simulink model "MIMO"  (R2019a)
settings: Solver=FixedStepAuto  StartTime=0.0  StopTime=inf  FixedStep=0.00001  RelTol=1e-3
libraries: dsparch4 x10
settings Model: NumberOfSteps=100  Creator=vardhah  LastModifiedBy=vardhah
settings DataIOCC: ReturnWorkspaceOutputs=off
settings DebuggingCC: UnderSpecifiedDimensionMsg=warning  ArithmeticOperatorsInVariantConditions=warning

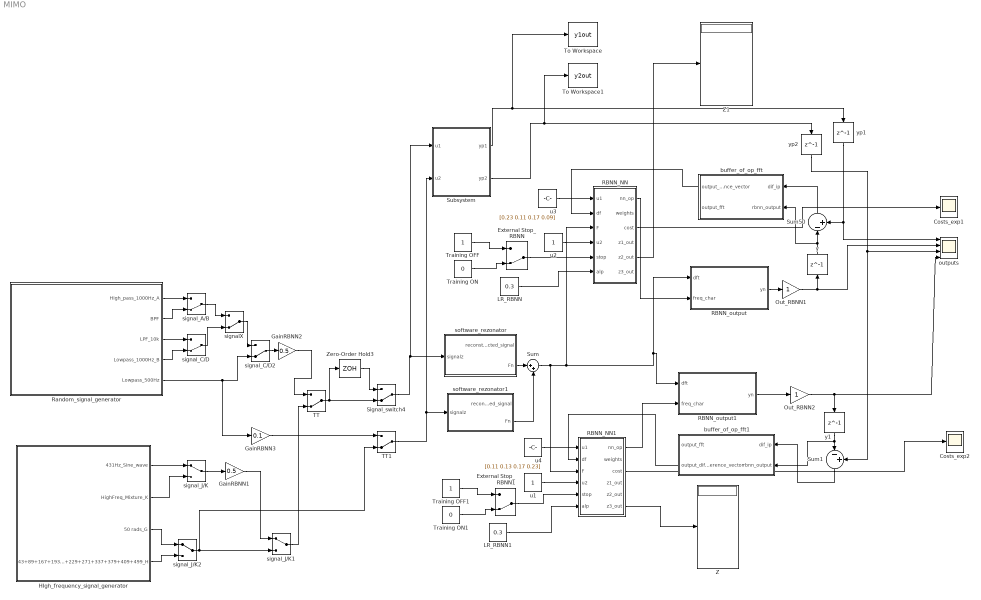
== system MIMO ==
  Costs_exp1 : Scope
  Costs_exp2 : Scope
  External Stop_RBNN : ManualSwitch  CurrentSetting=0
  External Stop_RBNN1 : ManualSwitch  CurrentSetting=0
  GainRBNN1 : Gain  Gain=0.5
  GainRBNN2 : Gain  Gain=0.5
  GainRBNN3 : Gain  Gain=0.1
  HIgh_frequency_signal_generator : Subsystem
  LR_RBNN : Constant  Value=0.3
  LR_RBNN1 : Constant  Value=0.3
  Out_RBNN1 : Gain
  Out_RBNN2 : Gain
  RBNN_NN : MATLAB Function  TreatAsAtomicUnit=on
  RBNN_NN1 : MATLAB Function  TreatAsAtomicUnit=on
  RBNN_output : MATLAB Function  TreatAsAtomicUnit=on
  RBNN_output1 : MATLAB Function  TreatAsAtomicUnit=on
  Random_signal_generator : Subsystem
  Signal_switch4 : ManualSwitch  CurrentSetting=0
  Subsystem : Subsystem
  Sum : Sum  Inputs=|++
  Sum1 : Sum  Inputs=|-+
  Sum50 : Sum  Inputs=|-+
  TT : ManualSwitch  CurrentSetting=0
  TT1 : ManualSwitch  CurrentSetting=0
  To Workspace : ToWorkspace  VariableName=y1out  SampleTime=-1
      settings: Save2DSignal=2-D array (concatenate along first dimension)
  To Workspace1 : ToWorkspace  VariableName=y2out  SampleTime=-1
      settings: Save2DSignal=2-D array (concatenate along first dimension)
  Training OFF : Constant
  Training OFF1 : Constant
  Training ON : Constant  Value=0
  Training ON1 : Constant  Value=0
  Z : Display
  Z1 : Display
  Zero-Order Hold3 : ZeroOrderHold  SampleTime=0.00001
  buffer_of_op_fft : MATLAB Function  TreatAsAtomicUnit=on
  buffer_of_op_fft1 : MATLAB Function  TreatAsAtomicUnit=on
  outputs : Scope  NumInputPorts=4
  signalX : ManualSwitch  CurrentSetting=0
  signal_A/B : ManualSwitch  CurrentSetting=0
  signal_C/D : ManualSwitch  CurrentSetting=0
  signal_C/D2 : ManualSwitch  CurrentSetting=0
  signal_J/K : ManualSwitch
  signal_J/K1 : ManualSwitch
  signal_J/K2 : ManualSwitch
  software_rezonator : MATLAB Function  TreatAsAtomicUnit=on
  software_rezonator1 : MATLAB Function  TreatAsAtomicUnit=on
  u1 : Constant
  u2 : Constant
  u3 : Constant  Value=[0.23 0.11 0.17 0.09]
  u4 : Constant  Value=[0.11 0.13 0.17 0.23]
  y : Delay  DelayLength=1  InitialCondition=0
  y1 : Delay  DelayLength=1  InitialCondition=0
  yp1 : Delay  DelayLength=1  InitialCondition=0
  yp2 : Delay  DelayLength=1  InitialCondition=0
  wires:
  software_rezonator/2(Fn) -> Sum/1
  RBNN_output/1(yn) -> Out_RBNN1/1
  External Stop_RBNN/1 -> RBNN_NN/5(stop)
  Training OFF/1 -> External Stop_RBNN/1
  Training ON/1 -> External Stop_RBNN/2
  Sum50/1 -> buffer_of_op_fft/1(dif_ip)
  TT/1 -> Zero-Order Hold3/1, Signal_switch4/2
  LR_RBNN/1 -> RBNN_NN/6(alp)
  Random_signal_generator/1(High_pass_1000Hz_A) -> signal_A/B/1
  signal_A/B/1 -> signalX/1
  signal_C/D/1 -> signalX/2
  signal_J/K1/1 -> TT/2
  Out_RBNN1/1 -> y/1, outputs/2
  HIgh_frequency_signal_generator/1(431Hz_Sine_wave) -> signal_J/K/1
  HIgh_frequency_signal_generator/2(HighFreq_Mixture_K) -> signal_J/K/2
  signal_J/K/1 -> GainRBNN1/1
  Signal_switch4/1 -> Subsystem/1(u1), software_rezonator/1(signalz)
  Random_signal_generator/3(LPF_10k) -> signal_C/D/1
  Random_signal_generator/2("BPF ") -> signal_A/B/2
  signalX/1 -> signal_C/D2/1
  Random_signal_generator/5(Lowpass_500Hz) -> GainRBNN3/1, signal_C/D2/2
  HIgh_frequency_signal_generator/3(50 rads_G) -> signal_J/K2/1
  HIgh_frequency_signal_generator/4(43+89+167+193+229+271+337+379+409+499_H) -> signal_J/K2/2
  GainRBNN1/1 -> signal_J/K1/1
  signal_C/D2/1 -> GainRBNN2/1
  GainRBNN2/1 -> TT/1
  Zero-Order Hold3/1 -> Signal_switch4/1
  u2/1 -> RBNN_NN/4(u2)
  LR_RBNN1/1 -> RBNN_NN1/6(alp)
  Training ON1/1 -> External Stop_RBNN1/2
  External Stop_RBNN1/1 -> RBNN_NN1/5(stop)
  Training OFF1/1 -> External Stop_RBNN1/1
  u1/1 -> RBNN_NN1/4(u2)
  software_rezonator1/2(Fn) -> Sum/2
  Random_signal_generator/4(Lowpass_1000Hz_B) -> signal_C/D/2
  TT1/1 -> Subsystem/2(u2), software_rezonator1/1(signalz)
  RBNN_NN/1(nn_op) -> RBNN_output/2(freq_char)
  Subsystem/1(yp1) -> To Workspace/1, yp1/1
  buffer_of_op_fft/1(output_difference_vector) -> RBNN_NN/2(df)
  RBNN_NN1/1(nn_op) -> RBNN_output1/2(freq_char)
  buffer_of_op_fft1/2(output_difference_vector) -> RBNN_NN1/2(df)
  y/1 -> buffer_of_op_fft/2(rbnn_output), Sum50/1
  yp1/1 -> outputs/1, Sum50/2
  RBNN_output1/1(yn) -> Out_RBNN2/1
  Out_RBNN2/1 -> y1/1, outputs/4
  Subsystem/2(yp2) -> To Workspace1/1, yp2/1
  yp2/1 -> outputs/3, Sum1/2
  RBNN_NN/3(cost) -> Costs_exp1/1
  Sum1/1 -> buffer_of_op_fft1/1(dif_ip)
  y1/1 -> buffer_of_op_fft1/2(rbnn_output), Sum1/1
  RBNN_NN1/3(cost) -> Costs_exp2/1
  signal_J/K2/1 -> TT1/2, signal_J/K1/2
  RBNN_NN/5(z2_out) -> Z1/1
  Sum/1 -> RBNN_NN1/3(F), RBNN_NN/3(F), RBNN_output/1(dft), RBNN_output1/1(dft)
  GainRBNN3/1 -> TT1/1
  RBNN_NN1/6(z3_out) -> Z/1
  u3/1 -> RBNN_NN/1(u1)
  u4/1 -> RBNN_NN1/1(u1)

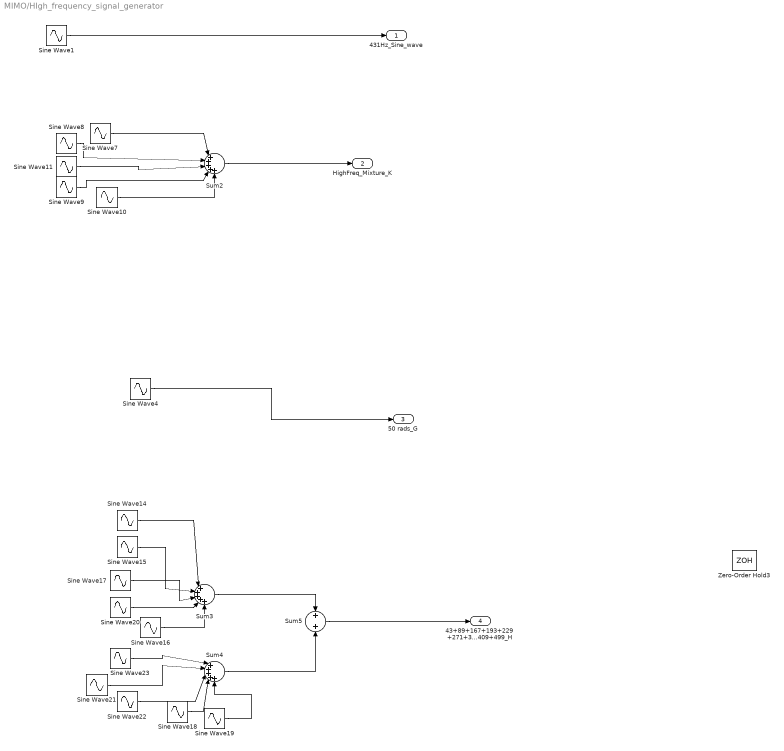
== system MIMO/HIgh_frequency_signal_generator ==
  Sine Wave1 : Sin  Amplitude=0.5  Frequency=431  SampleTime=0
  Sine Wave10 : Sin  Amplitude=2  Frequency=47000  SampleTime=0
  Sine Wave11 : Sin  Amplitude=2  Frequency=30637  SampleTime=0
  Sine Wave14 : Sin  Amplitude=0.1  Frequency=43  SampleTime=0
  Sine Wave15 : Sin  Amplitude=0.1  Frequency=89  SampleTime=0
  Sine Wave16 : Sin  Amplitude=0.1  Frequency=229  SampleTime=0
  Sine Wave17 : Sin  Amplitude=0.1  Frequency=167  SampleTime=0
  Sine Wave18 : Sin  Amplitude=0.1  Frequency=409  SampleTime=0
  Sine Wave19 : Sin  Amplitude=0.1  Frequency=499  SampleTime=0
  Sine Wave20 : Sin  Amplitude=0.1  Frequency=193  SampleTime=0
  Sine Wave21 : Sin  Amplitude=0.1  Frequency=337  SampleTime=0
  Sine Wave22 : Sin  Amplitude=0.1  Frequency=379  SampleTime=0
  Sine Wave23 : Sin  Amplitude=0.1  Frequency=271  SampleTime=0
  Sine Wave4 : Sin  Amplitude=0.5  Frequency=50  SampleTime=0
  Sine Wave7 : Sin  Amplitude=2  Frequency=28230  SampleTime=0
  Sine Wave8 : Sin  Amplitude=2  Frequency=33927  SampleTime=0
  Sine Wave9 : Sin  Amplitude=0  Frequency=53787  SampleTime=0
  Sum2 : Sum  Inputs=|+++++
  Sum3 : Sum  Inputs=|+++++
  Sum4 : Sum  Inputs=|+++++
  Sum5 : Sum
  Zero-Order Hold3 : ZeroOrderHold  SampleTime=0.00001
  431Hz_Sine_wave : Outport
  HighFreq_Mixture_K : Outport  Port=2
  50 rads_G : Outport  Port=3
  43+89+167+193+229+271+337+379+409+499_H : Outport  Port=4
  wires:
  Sine Wave9/1 -> Sum2/4
  Sine Wave7/1 -> Sum2/1
  Sine Wave10/1 -> Sum2/5
  Sine Wave8/1 -> Sum2/2
  Sine Wave11/1 -> Sum2/3
  Sine Wave1/1 -> 431Hz_Sine_wave/1
  Sum2/1 -> HighFreq_Mixture_K/1
  Sine Wave23/1 -> Sum4/1
  Sine Wave17/1 -> Sum3/3
  Sine Wave22/1 -> Sum4/3
  Sine Wave18/1 -> Sum4/4
  Sine Wave19/1 -> Sum4/5
  Sine Wave20/1 -> Sum3/4
  Sine Wave14/1 -> Sum3/1
  Sine Wave15/1 -> Sum3/2
  Sine Wave21/1 -> Sum4/2
  Sine Wave16/1 -> Sum3/5
  Sum4/1 -> Sum5/2
  Sum3/1 -> Sum5/1
  Sine Wave4/1 -> 50 rads_G/1
  Sum5/1 -> 43+89+167+193+229+271+337+379+409+499_H/1

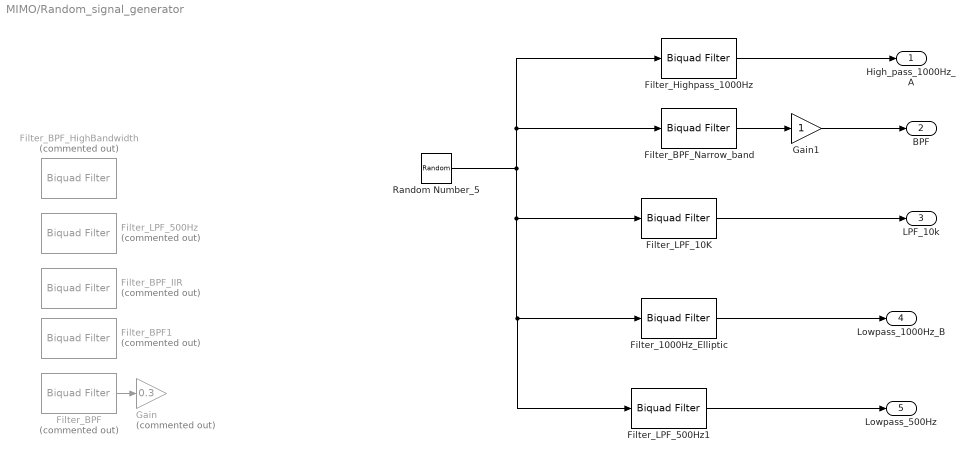
== system MIMO/Random_signal_generator ==
  Filter_1000Hz_Elliptic : dsparch4/Biquad Filter  Tag=BlockMethodSubSystem  FilterSource=Dialog parameters  CoeffSource=Specify via dialog  FilterObject=BQF  IIRFiltStruct=Direct form II  BiQuadCoeffs=[1 -1.97632274641133088 1 1 -1.97939835930391728 0.996447647782941925;1 -1.97278944538463175 1 1 -1.97237302925889701 0.987301248342435933;1 -1.95955871016892758 1 1 -1.96235771308246942 0.972660421241710926;1 -1.88453112329299022 1 1 -1.95007892273323602 0.954154972801176005;1 1 0 1 -0.971866907997287366 0]  ScaleValues=[0.156742012624585314;0.548618699418480849;0.254757160374388947;0.035299988916345823;0.064621492680459483;1]  IC=0  ICnum=0  ICden=0  a0Flag=Warning  optimizeScaleValues=on  ScaleValueMode=Specify via input port (g)  InputProcessing=Columns as channels (frame based)  roundingMode=Floor  overflowMode=off  scaleValueFracLength=14  denProdOutputFracLength=30  denAccumFracLength=30  secondMemoryFracLength=15
      settings: SourceProductName=DSP System Toolbox
  Filter_BPF : dsparch4/Biquad Filter  Tag=BlockMethodSubSystem  Commented=on  FilterSource=Dialog parameters  CoeffSource=Specify via dialog  FilterObject=BQF  IIRFiltStruct=Direct form II  BiQuadCoeffs=[1 -1.97761973100167809 1 1 1.57870632394964705 0.920020418344257962;1 1.77936221516677162 1 1 -1.93552590907125399 0.972267372386662942;1 -1.98005309158266063 1 1 1.47905907116838886 0.778576723939160997;1 1.80228019362095471 1 1 -1.8859717379982055 0.919695136491283316;1 -1.98441806776151775 1 1 -1.84268162877499142 0.871961176321420783;1 1.84402260102226045 1 1 1.40847943705151635 0.659380286133449012;1 -1.98978059787965811 1 1 -1.8064582693224005 0.83068683784082864;1 1.89644656024463654 1 1 1.35993304577530516 0.561880786756156714;1 -1.99493211957147487 1 1 -1.77859151837716212 0.798148234549097224;1 1.94803425022672294 1 1 1.32826652221219343 0.488041230314220198;1 -1.99864670422051782 1 1 -1.76078971043777521 0.777037775895594751;1 1.98600294595924809 1 1 1.31027557706720854 0.441399359096070587;1 0 -1 1 -0.225108906907530854 -0.5721944072401276]  ScaleValues=[0.94218659324992049;0.94218659324992049;0.896412139345828973;0.896412139345828973;0.858240609492223139;0.858240609492223139;0.827592837896180988;0.827592837896180988;0.804900029269587591;0.804900029269587591;0.790860073802791552;0.790860073802791552;0.786097203620063856;1]  IC=0  ICnum=0  ICden=0  a0Flag=Warning  optimizeScaleValues=on  ScaleValueMode=Specify via input port (g)  InputProcessing=Columns as channels (frame based)  roundingMode=Floor  overflowMode=off  scaleValueFracLength=14  denProdOutputFracLength=30  denAccumFracLength=30  secondMemoryFracLength=15
      settings: SourceProductName=DSP System Toolbox
  Filter_BPF1 : dsparch4/Biquad Filter  Tag=BlockMethodSubSystem  Commented=on  FilterSource=Dialog parameters  CoeffSource=Specify via dialog  FilterObject=BQF  IIRFiltStruct=Direct form II  BiQuadCoeffs=[1 -1.87162275664653865 1 1 0.0151789185122153114 0.97249456913610377;1 0.107053815110264378 1 1 -1.8502247355910888 0.989791248656434752;1 -1.87399697860168635 1 1 0.0292079264951085604 0.918601061350948767;1 0.126268370493222148 1 1 -1.83332118307014369 0.969469007130600025;1 -1.87872867044463465 1 1 0.0569157635014451713 0.864412592104086164;1 0.165552966551231862 1 1 -1.81812689818783735 0.948927647744083225;1 -1.88577621884367863 1 1 -1.8041786729911804 0.927783166166077922;1 0.226641198999771337 1 1 0.097812015244096856 0.808034579697935573;1 -1.89505605753386197 1 1 -1.79101562259146441 0.90569591944563943;1 0.312164718875241609 1 1 0.151460725355784309 0.74780602813150221;1 -1.90641512361342702 1 1 -1.77818269270842544 0.882393193837985756;1 0.425602178644961193 1 1 0.217201621241827264 0.682338033780143238;1 -1.91959159061561468 1 1 -1.76525054298619066 0.857713442273093762;1 0.571003956082658304 1 1 0.293797239380520436 0.610677959292126982;1 -1.93416461417083374 1 1 -1.75186392449751338 0.831683197854011347;1 0.752181231021604835 1 1 0.379002473503964599 0.532637148822792561;1 -1.94949927666361944 1 1 -1.73783535618849294 0.804640333462611768;1 0.970805587395975667 1 1 0.469112491907584639 0.449311075928955861;1 -1.96470348628740155 1 1 -1.72330128044392006 0.777413997776565835;1 1.22267124909860003 1 1 0.558648874108559568 0.363760367241365734;1 -1.97862850586430206 1 1 -1.70893825597331972 0.751545290116931608;1 1.49181652406040532 1 1 0.640463654393117032 0.28166537946727177;1 -1.98995570459027227 1 1 -1.6961607248116688 0.729445514574812215;1 1.74459803428737614 1 1 0.706553803150463011 0.211486877483081787;1 -1.9973994069383596 1 1 -1.68705750203480132 0.71421185466085324;1 1.93071581234363698 1 1 0.749581571245088285 0.163359895205374334;1 0 -1 1 -0.45960409018619558 -0.321805205203900269]  ScaleValues=[0.947999620287395151;0.947999620287395151;0.929748841120282554;0.929748841120282554;0.910904712958650942;0.910904712958650942;0.890940239596866634;0.890940239596866634;0.869397912584866428;0.869397912584866428;0.845915862145971476;0.845915862145971476;0.820293089159258471;0.820293089159258471;0.792605314952226081;0.792605314952226081;0.763377121832675587;0.763377121832675587;0.733791113440760645;0.733791113440760645;0.705857588574427597;0.705857588574427597;0.682382892583755729;0.682382892583755729;0.666528818859254413;0.666528818859254413;0.660902602601950107;1]  IC=0  ICnum=0  ICden=0  a0Flag=Warning  optimizeScaleValues=on  ScaleValueMode=Specify via input port (g)  InputProcessing=Columns as channels (frame based)  roundingMode=Floor  overflowMode=off  scaleValueFracLength=14  denProdOutputFracLength=30  denAccumFracLength=30  secondMemoryFracLength=15
      settings: SourceProductName=DSP System Toolbox
  Filter_BPF_HighBandwidth : dsparch4/Biquad Filter  Tag=BlockMethodSubSystem  Commented=on  FilterSource=Dialog parameters  CoeffSource=Specify via dialog  FilterObject=BQF  IIRFiltStruct=Direct form II  BiQuadCoeffs=[1 1.7667446216002245 1 1 1.58209736682341973 0.930966785022698806;1 -1.34582318986797533 1 1 -0.992426842776809148 0.899039050324202504;1 1.79067372195770425 1 1 -0.914728053198516244 0.716995181890824007;1 -1.40612551986482726 1 1 1.48400011430024925 0.801184577292333389;1 1.83602350074132281 1 1 -0.851515418032590565 0.547239550845750156;1 -1.52433209950181525 1 1 1.39252668353121223 0.674238480546462959;1 1.89581887946284833 1 1 1.29703137445886307 0.544576166858187882;1 -1.6885603993121634 1 1 -0.786012220300839282 0.382455837322811409;1 1.95573661837008239 1 1 1.19088356295662234 0.413755766632151967;1 -1.86350238128714696 1 1 -0.705134792353248718 0.2271878178236309;1 1.99461273858363541 1 1 1.09074964949811615 0.306078291590546059;1 -1.98303965563176376 1 1 -0.619529972182138677 0.110169074458665181]  ScaleValues=[0.832448302986908639;0.832448302986908639;0.765789381177460982;0.765789381177460982;0.705208129127222416;0.705208129127222416;0.651112560595629053;0.651112560595629053;0.608221202899987934;0.608221202899987934;0.583850801160644806;0.583850801160644806;1]  IC=0  ICnum=0  ICden=0  a0Flag=Warning  optimizeScaleValues=on  ScaleValueMode=Specify via input port (g)  InputProcessing=Columns as channels (frame based)  roundingMode=Floor  overflowMode=off  scaleValueFracLength=14  denProdOutputFracLength=30  denAccumFracLength=30  secondMemoryFracLength=15
      settings: SourceProductName=DSP System Toolbox
  Filter_BPF_IIR : dsparch4/Biquad Filter  Tag=BlockMethodSubSystem  Commented=on  FilterSource=Dialog parameters  CoeffSource=Specify via dialog  FilterObject=BQF  IIRFiltStruct=Direct form II  BiQuadCoeffs=[1 -1.149490264419329 1 1 -0.626392877901499556 0.920117434054556482;1 0.646230741294248623 1 1 0.0366640948662285138 0.915703951328018961;1 -1.34532900218332485 1 1 -0.519313485606232472 0.780807553044220226;1 0.918145007146928704 1 1 -0.0338871305922869778 0.772019964264916481;1 -1.83355458637284285 1 1 -0.358020160863192105 0.687764548138794729;1 1.69599580965141206 1 1 -0.17451489355262309 0.683094681391207548]  ScaleValues=[0.380605401112502073;0.380605401112502073;0.290603776410566172;0.290603776410566172;0.185292453644045008;0.185292453644045008;1]  IC=0  ICnum=0  ICden=0  a0Flag=Warning  optimizeScaleValues=on  ScaleValueMode=Specify via input port (g)  InputProcessing=Columns as channels (frame based)  roundingMode=Floor  overflowMode=off  scaleValueFracLength=14  denProdOutputFracLength=30  denAccumFracLength=30  secondMemoryFracLength=15
      settings: SourceProductName=DSP System Toolbox
  Filter_BPF_Narrow_band : dsparch4/Biquad Filter  Tag=BlockMethodSubSystem  FilterSource=Dialog parameters  CoeffSource=Specify via dialog  FilterObject=BQF  IIRFiltStruct=Direct form II  BiQuadCoeffs=[1 0.62090288091487722 1 1 0.531418224661316274 0.980919730652416666;1 0.123603302701670317 1 1 0.212906146103049365 0.980314531399748446;1 0.646038601655443578 1 1 0.517597147874857333 0.941099448368431624;1 0.0957486348882208987 1 1 0.211835114073677666 0.93930845670321006;1 0.711459208664077192 1 1 0.494162772086789159 0.895904757499573212;1 0.0218734686284944163 1 1 0.218844224698679646 0.893061304454884519;1 0.877256774030408248 1 1 0.450892485812207533 0.84715521652707737;1 -0.17476459239363229 1 1 0.245263071402918309 0.844050263048180871;1 1.47045699040561728 1 1 0.381616270905086485 0.810187489215232537;1 -1.01162752930746769 1 1 0.302620729086598206 0.808716245866266337]  ScaleValues=[0.644925573949283848;0.644925573949283848;0.594784290548588279;0.594784290548588279;0.499322257310351236;0.499322257310351236;0.34838267808004042;0.34838267808004042;0.155186261234775053;0.155186261234775053;1]  IC=0  ICnum=0  ICden=0  a0Flag=Warning  optimizeScaleValues=on  ScaleValueMode=Specify via input port (g)  InputProcessing=Columns as channels (frame based)  roundingMode=Floor  overflowMode=off  scaleValueFracLength=14  denProdOutputFracLength=30  denAccumFracLength=30  secondMemoryFracLength=15
      settings: SourceProductName=DSP System Toolbox
  Filter_Highpass_1000Hz : dsparch4/Biquad Filter  Tag=BlockMethodSubSystem  FilterSource=Dialog parameters  CoeffSource=Specify via dialog  FilterObject=BQF  IIRFiltStruct=Direct form II  BiQuadCoeffs=[1 -1.9832348135082305 1 1 -1.92871230100246671 0.962722433368264241;1 -1.98583197848424597 1 1 -1.86448430214602556 0.894880266245439038;1 -1.99020937824944788 1 1 -1.81348943480495617 0.839000119522318677;1 -1.99498360843622446 1 1 -1.77690733715439997 0.797591087467987903;1 -1.99863653257112794 1 1 -1.75501257669195576 0.772196386514157451;1 -1 0 1 -0.873867637211059756 0]  ScaleValues=[0.976953385016072651;0.943181897451958351;0.915362881516173843;0.894746706112661938;0.882102920451765637;0.936933818605529933;1]  IC=0  ICnum=0  ICden=0  a0Flag=Warning  optimizeScaleValues=on  ScaleValueMode=Specify via input port (g)  InputProcessing=Columns as channels (frame based)  roundingMode=Floor  overflowMode=off  scaleValueFracLength=14  denProdOutputFracLength=30  denAccumFracLength=30  secondMemoryFracLength=15
      settings: SourceProductName=DSP System Toolbox
  Filter_LPF_10K : dsparch4/Biquad Filter  Tag=BlockMethodSubSystem  FilterSource=Dialog parameters  CoeffSource=Specify via dialog  FilterObject=BQF  IIRFiltStruct=Direct form II  BiQuadCoeffs=[1 2 1 1 -0.612485417634850315 0.975058739649728001;1 2 1 1 -0.698043577421757266 0.925601996299419083;1 2 1 1 -0.874476472259565263 0.875096533006947785;1 2 1 1 -1.12129625964924906 0.823722261210925066;1 2 1 1 -1.39397155012670271 0.77557292582325299;1 2 1 1 -1.61651585106992179 0.739432707187852145;1 1 0 1 -0.851908249730889411 0]  ScaleValues=[0.340643330503719421;0.306889604719415399;0.250155015186845686;0.175606500390419001;0.0954003439241375567;0.0307292140294825808;0.0740458751345553223;1]  IC=0  ICnum=0  ICden=0  a0Flag=Warning  optimizeScaleValues=on  ScaleValueMode=Specify via input port (g)  InputProcessing=Columns as channels (frame based)  roundingMode=Floor  overflowMode=off  scaleValueFracLength=14  denProdOutputFracLength=30  denAccumFracLength=30  secondMemoryFracLength=15
      settings: SourceProductName=DSP System Toolbox
  Filter_LPF_500Hz : dsparch4/Biquad Filter  Tag=BlockMethodSubSystem  Commented=on  FilterSource=Dialog parameters  CoeffSource=Specify via dialog  FilterObject=BQF  IIRFiltStruct=Direct form II  BiQuadCoeffs=[1 -1.99378181081805117 1 1 -1.98902831364610422 0.9935124525991188;1 -1.99333638931724444 1 1 -1.97523846334044983 0.979918343946878045;1 -1.99230894289473004 1 1 -1.95902587969734232 0.964154555843562355;1 -1.99032724021591334 1 1 -1.93837876272327003 0.944275888371317706;1 -1.98644110500488824 1 1 -1.91073325330636345 0.917824821659265599;1 -1.97784207285711422 1 1 -1.87346681472727061 0.882295849747020466;1 -1.95323474003079056 1 1 -1.82673924270665844 0.837830591019173787;1 -1.8251127117585888 1 1 -1.78083961390105383 0.794192376902756902;1 1 0 1 -0.880096604509032043 0]  ScaleValues=[0.721132603368186742;0.702304025434590584;0.6668363107986508;0.609663196407451258;0.523019638064808889;0.398459430018688054;0.237170675835394501;0.0763506778335484859;0.0599516977454839714;1]  IC=0  ICnum=0  ICden=0  a0Flag=Warning  optimizeScaleValues=on  ScaleValueMode=Specify via input port (g)  InputProcessing=Columns as channels (frame based)  roundingMode=Floor  overflowMode=off  scaleValueFracLength=14  denProdOutputFracLength=30  denAccumFracLength=30  secondMemoryFracLength=15
      settings: SourceProductName=DSP System Toolbox
  Filter_LPF_500Hz1 : dsparch4/Biquad Filter  Tag=BlockMethodSubSystem  FilterSource=Dialog parameters  CoeffSource=Specify via dialog  FilterObject=BQF  IIRFiltStruct=Direct form II  BiQuadCoeffs=[1 -1.99378181081805117 1 1 -1.98902831364610422 0.9935124525991188;1 -1.99333638931724444 1 1 -1.97523846334044983 0.979918343946878045;1 -1.99230894289473004 1 1 -1.95902587969734232 0.964154555843562355;1 -1.99032724021591334 1 1 -1.93837876272327003 0.944275888371317706;1 -1.98644110500488824 1 1 -1.91073325330636345 0.917824821659265599;1 -1.97784207285711422 1 1 -1.87346681472727061 0.882295849747020466;1 -1.95323474003079056 1 1 -1.82673924270665844 0.837830591019173787;1 -1.8251127117585888 1 1 -1.78083961390105383 0.794192376902756902;1 1 0 1 -0.880096604509032043 0]  ScaleValues=[0.721132603368186742;0.702304025434590584;0.6668363107986508;0.609663196407451258;0.523019638064808889;0.398459430018688054;0.237170675835394501;0.0763506778335484859;0.0599516977454839714;1]  IC=0  ICnum=0  ICden=0  a0Flag=Warning  optimizeScaleValues=on  ScaleValueMode=Specify via input port (g)  InputProcessing=Columns as channels (frame based)  roundingMode=Floor  overflowMode=off  scaleValueFracLength=14  denProdOutputFracLength=30  denAccumFracLength=30  secondMemoryFracLength=15
      settings: SourceProductName=DSP System Toolbox
  Gain : Gain  Commented=on  Gain=0.3
  Gain1 : Gain
  Random Number_5 : RandomNumber  Variance=0.5  SampleTime=0.00001
  High_pass_1000Hz_A : Outport
  "BPF " : Outport  Port=2
  LPF_10k : Outport  Port=3
  Lowpass_1000Hz_B : Outport  Port=4
  Lowpass_500Hz : Outport  Port=5
  wires:
  Filter_Highpass_1000Hz/1 -> High_pass_1000Hz_A/1
  Filter_1000Hz_Elliptic/1 -> Lowpass_1000Hz_B/1
  Filter_BPF/1 -> Gain/1
  Gain1/1 -> "BPF "/1
  Filter_LPF_10K/1 -> LPF_10k/1
  Random Number_5/1 -> Filter_LPF_500Hz1/1, Filter_1000Hz_Elliptic/1, Filter_LPF_10K/1, Filter_BPF_Narrow_band/1, Filter_Highpass_1000Hz/1
  Filter_BPF_Narrow_band/1 -> Gain1/1
  Filter_LPF_500Hz1/1 -> Lowpass_500Hz/1

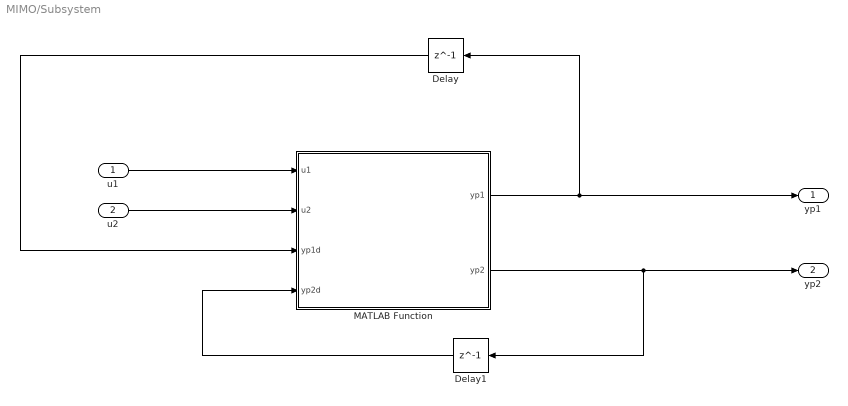
== system MIMO/Subsystem ==
  u1 : Inport
  u2 : Inport  Port=2
  Delay : Delay  DelayLength=1  InitialCondition=0
  Delay1 : Delay  DelayLength=1  InitialCondition=0
  MATLAB Function : MATLAB Function  TreatAsAtomicUnit=on
  yp1 : Outport
  yp2 : Outport  Port=2
  wires:
  u1/1 -> MATLAB Function/1(u1)
  MATLAB Function/2(yp2) -> yp2/1, Delay1/1
  u2/1 -> MATLAB Function/2(u2)
  MATLAB Function/1(yp1) -> Delay/1, yp1/1
  Delay/1 -> MATLAB Function/3(yp1d)
  Delay1/1 -> MATLAB Function/4(yp2d)

== matlab function MIMO/Subsystem/MATLAB Function ==
  data: u1 input; yp1 output; u2 input; yp2 output; yp1d input; yp2d input
function [yp1,yp2] = fcn(u1,u2, yp1d, yp2d)



yp1 = u2*(u2-0.8)*(u2+0.5)+(yp2d)/(1+yp2d);
yp2 = -u1^2+(yp2d*yp1d/(1+yp1d));


%yp1 = u1+(yp1d)/(1+yp2d^2);
%yp2 = u2+(yp2d*yp1d/(1+yp2d^2));

== matlab function MIMO/RBNN_NN ==
  settings: sampleTime=0.01
  data: u1 input; df input; F input; u2 input; nn_op output; weights output; cost output; z1_out output; stop input; alp input; z2_out output; z3_out output
function [nn_op,weights,cost,z1_out,z2_out,z3_out]  = NN(u1,df,F,u2,stop,alp)

persistent w1 w2 w3;
persistent vy;
persistent g1 g2 g3;
persistent itr;
persistent J;
persistent del_w1 del_w2 del_w3;
persistent mult1 mult2 mult3;
persistent memory_alloc_flag;
persistent n;

%%
%%%%%%----------------------------------------------------------------------------%%%%%
%Hyper-parameter & other tunable part of code

M=4;   %declare batch size of training (It will also be equal to number of input in our case as we are using DFT)
E=1;    % size of external associative input

%layer declaration
layer_1=32;
layer_2=32;
layer_3=8;       % Output layer must match with number of rezonators declared in rezonator function

%learning rate. Currently reading from input pin 
alpha = alp;

%others
input_layer =M+E;       %layer_0
output_layer=layer_3;

% weight Intialisation 
if isempty(w1)
       w1=randn(input_layer,layer_1)*0.1;
end
if isempty(w2)
       w2=randn(layer_1,layer_2)*0.1;
end
if isempty(w3)
       w3=randn(layer_2,layer_3)*0.1;
end

%%%%%---------------------------------------------------------------------------------%%%%%

%%

%synchronising clock
if isempty(n)
        n = 0; end
n=n+1;

%%
%Allocation of variables that will be used during runtime( one time execution code) 
if isempty(memory_alloc_flag)
        memory_alloc_flag = 0; 
end
if isempty(mult1)
       mult1=zeros(layer_1,layer_1*input_layer); 
end
if isempty(mult2)
       mult2=zeros(layer_2,layer_1*layer_2); 
end
if isempty(mult3)
       mult3=zeros(layer_3,layer_2*layer_3); 
end
if isempty(vy)
       vy=zeros(input_layer,M); 
end

if memory_alloc_flag==0
 %write memory allocation for looped code here.It runs once and store it in memory.  
 mult1=[];
 mult2=[];
 mult3=[];
  for iteration =1:layer_1
   mult1=[mult1;[zeros(1,(iteration-1)*input_layer) ones(1,input_layer) zeros(1,(layer_1-iteration)*input_layer)]];
  end
  for iterate=1:layer_2
   mult2=[mult2;[zeros(1,(iterate-1)*layer_1) ones(1,layer_1) zeros(1,(layer_2-iterate)*layer_1)]];
  end
  for iterate=1:layer_3
   mult3=[mult3;[zeros(1,(iterate-1)*layer_2) ones(1,layer_2) zeros(1,(layer_3-iterate)*layer_2)]];
  end
 
 for k= 1:input_layer
    for j = 1:M 
        if k<=(M/2)+1 && k>=1
            vy(k,j)=(1/M)*cos(pi*(M-j)*(k-1)/(M/2));
        elseif k<=M && k>=(M/2)+1
            vy(k,j)=-(1/M)*sin(pi*(M-j)*(k-1)/(M/2));
        elseif k>M
            vy(k,j)=0;     
        end
    end
 end
 memory_alloc_flag=1; 
end

%%
%============All other Initiaisation =========================>

%Initialisation of delta of weight storage
if isempty(del_w1)
    del_w1=zeros(1,input_layer*layer_1);
end
if isempty(del_w2)
    del_w2=zeros(1,layer_2*layer_1);
end
if isempty(del_w3)
    del_w3=zeros(1,layer_2*layer_3);
end

%Intialising iteration number & cost value. 
if isempty(itr)
    itr=0;
end
if isempty(J)
    J=0;
end


%gradient initialisation(in matrix form)
if isempty(g1)
    g1= zeros(M,input_layer*layer_1);   
end
if isempty(g2)
    g2= zeros(M,layer_1*layer_2);   
end
if isempty(g3)
    g3= zeros(M,layer_3*layer_2);   
end

%%
%Input vector creation code block
%x_in = [real(u1(1:(size(u1,2)/2)+1)) imag(u1(1:(size(u1,2)/2)-1))];
%v=transpose([x_in transpose(u2)]);

v=transpose([u1' transpose(u2)]);

%%
%RBNN core vectorised algorithm implementation 

%--------------->forward propogation ------------>

z1=w1'*v ;
%a1=(1./(1+exp(-z1)));
%an1=(a1-0.5);
a1=max(z1,0)+0.1*min(0,z1);
z2=w2'*a1 ;
%z2=w2'*an1 ;
%a2=(1./(1+exp(-z2)));
%an2=(a2-0.5);
a2=max(z2,0)+0.1*min(0,z2);
%z3=w3'*an2 ;
z3=w3'*a2 ;
a3=(1./(1+exp(-z3)));
an3=(a3-0.5)*10;

%-------------> Backward Propogation -------->

%calculation of Nv:
da3_z3=a3.*(1-a3)*10;
dn_a2=w3'.*repmat(da3_z3,1,layer_2);
%da2_z2=a2.*(1-a2);
da2_z2=(1*(a2>=0) + 0.1*((a2>=0)==0));
dn_z2= dn_a2.* repmat(transpose(da2_z2),output_layer,1);
dn_a1=dn_z2*w2';
%da1_z1=a1.*(1-a1); 
da1_z1=(1*(a1>=0) + 0.1*((a1>=0)==0));
dn_z1=dn_a1.*repmat(transpose(da1_z1),output_layer,1);
dn_v=dn_z1*w1';   %"This is Nv" 

%calculation of aD, A & B 
aD=transpose(F)*dn_v*vy;
A=[aD;eye(M-1) zeros(M-1,1)];
B=[transpose(F) ; zeros(M-1,size(F,1))]; 

%calculation of Nw(diff of N(v,w) wrt each weights)
dIn_3= da3_z3*transpose(a2);
dn_w3=repmat(dIn_3,1,layer_3).* mult3;

dIn_2= da2_z2*transpose(a1);
da2_w2=repmat(dIn_2,1,layer_2).* mult2;
dn_w2=dn_a2*da2_w2;

dIn_1= da1_z1*transpose(v);
da1_w1= repmat(dIn_1,1,layer_1).*mult1;
dn_w1=dn_a1*da1_w1;

%gradient updation
g3=A*g3+B*dn_w3;
g2=A*g2+B*dn_w2;
g1=A*g1+B*dn_w1;

%Training & updation only once in a batch(batch size=M,n=Overall counter) 
if mod(n,M)==0 && stop==0
    del_w1 =alpha*df*1*g1/M ;
    del_w2 =alpha*df*1*g2/M ;
    del_w3 =alpha*df*1*g3/M ;
    del_w_reshaped1= reshape(del_w1,[input_layer,layer_1]);
    del_w_reshaped2= reshape(del_w2,[layer_1,layer_2]);
    del_w_reshaped3= reshape(del_w3,[layer_2,layer_3]);
    w1=w1+ del_w_reshaped1;
    w2=w2+ del_w_reshaped2;
    w3=w3+ del_w_reshaped3; 
    itr=itr+1;
    J= sum(df.^2,'all')/(2*M);
end

%For logging & visulisation purpose
cost=J;
weights=w1;
z1_out=z1;
z2_out=z2;
z3_out=z3;

%NN output assignment
nn_op=an3;


end

== matlab function MIMO/buffer_of_op_fft ==
  data: output_difference_vector output size=[1,4]; output_fft output size=[1,4]; dif_ip input; rbnn_output input
function [output_difference_vector,output_fft] = difBuffer(dif_ip,rbnn_output)                      

 sz=4;                       % size of the dft 
 
 persistent a;
 persistent b;
 if isempty(b)
  b= zeros(1,sz);
 end
 if isempty(a)
  a= zeros(1,sz);
 end
 
 
  a= circshift(a,1);
  a(1)=dif_ip;
  b= circshift(b,1);
  b(1)=rbnn_output;

 output_difference_vector=a; 
 output_fft=1/sz*fft(b); 
end

== matlab function MIMO/software_rezonator1 ==
  data: signalz input; reconstructed_signal output; Fn output size=8
function [reconstructed_signal,Fn]   = rezonator(signalz)

persistent numberofrezonator;
persistent g c bfr_rezo_sm aft_delay dft_out;
persistent out signal_dif;
persistent n;
persistent memory_alloc_flag;


%assign the number of rezonator here. For configuring it for higher order
%rezonator  we need to change (1) 'numberofrezonaotor' variable
if isempty(numberofrezonator)
        numberofrezonator = 8;   %here 16 parallel rezonators
end
N=8;
%Initialisation of memory allocations/variables ====> 
if isempty(memory_alloc_flag)
        memory_alloc_flag = 0; 
end
if isempty(g)
       g=zeros(numberofrezonator,numberofrezonator,'like',0i); 
end
if isempty(c)
       c=zeros(numberofrezonator,numberofrezonator,'like',0i); 
end
if memory_alloc_flag==0
 for i=0:numberofrezonator-1
  for j= 0:numberofrezonator-1
   g(i+1,j+1)=1/numberofrezonator*(exp(-1i*2*pi*i*j/numberofrezonator));
   c(i+1,j+1)=(exp(1i*2*pi*i*j/numberofrezonator));
  end 
 end
 memory_alloc_flag=1;
end


%Initialisation of variables  =====> 
if isempty(n)
        n = 0;   
end 
if isempty(out)
  out=0+0i;
end
if isempty(signal_dif)
  signal_dif=0+0i;
end
if isempty(bfr_rezo_sm)
  bfr_rezo_sm=repmat(0+0i,numberofrezonator,1);
end
if isempty(aft_delay)
  aft_delay=repmat(0+0i,numberofrezonator,1);
end
if isempty(dft_out)
  dft_out=repmat(0+0i,numberofrezonator,1);
end

%creating cycle of rotation for selection of correct column of g & c.
cycle=mod(n,numberofrezonator);

%resonator core -----------------------------> 
dft_out=c(:,cycle+1).*aft_delay;
out= sum(dft_out,1);
signal_dif=signalz-out;
bfr_rezo_sm=g(:,cycle+1).*signal_dif;

%counting the counter
n=n+1;

% output assignment ------------------>
reconstructed_signal=out;
dft=aft_delay; 
%N=size(dft,1);
a=1:1:N/2-1;
b=N/2+1:1:N-1;
dft_trans=transpose(dft);
Fn=5*transpose([real(dft_trans(1)) 2*(real(dft_trans(2:N/2)).*cos(2*pi*a*n/N)-imag(dft_trans(2:N/2)).*sin(2*pi*a*n/N)) -1^n*real(dft_trans(N/2+1)) -2*(imag(dft_trans(N/2+2:N)).*cos(2*pi*b*n/N)+real(dft_trans(N/2+2:N)).*sin(2*pi*b*n/N))]);
%--------output assignment over----------<

%final updation of buffer ------>>>>>>>>>>>>
aft_delay= aft_delay+bfr_rezo_sm; 
end

== matlab function MIMO/RBNN_NN1 ==
  settings: sampleTime=0.01
  data: u1 input; df input; F input; u2 input; nn_op output; weights output; cost output; z1_out output; stop input; alp input; z2_out output; z3_out output
function [nn_op,weights,cost,z1_out,z2_out,z3_out]  = NN(u1,df,F,u2,stop,alp)

persistent w1 w2 w3;
persistent vy;
persistent g1 g2 g3;
persistent itr;
persistent J;
persistent del_w1 del_w2 del_w3;
persistent mult1 mult2 mult3;
persistent memory_alloc_flag;
persistent n;

%%
%%%%%%----------------------------------------------------------------------------%%%%%
%Hyper-parameter & other tunable part of code

M=4;   %declare batch size of training (It will also be equal to number of input in our case as we are using DFT)
E=1;    % size of external associative input

%layer declaration
layer_1=32;
layer_2=32;
layer_3=8;       % Output layer must match with number of rezonators declared in rezonator function

%learning rate. Currently reading from input pin 
alpha = alp;

%others
input_layer =M+E;       %layer_0
output_layer=layer_3;

% weight Intialisation 
if isempty(w1)
       w1=randn(input_layer,layer_1)*0.1;
end
if isempty(w2)
       w2=randn(layer_1,layer_2)*0.1;
end
if isempty(w3)
       w3=randn(layer_2,layer_3)*0.1;
end

%%%%%---------------------------------------------------------------------------------%%%%%

%%

%synchronising clock
if isempty(n)
        n = 0; end
n=n+1;

%%
%Allocation of variables that will be used during runtime( one time execution code) 
if isempty(memory_alloc_flag)
        memory_alloc_flag = 0; 
end
if isempty(mult1)
       mult1=zeros(layer_1,layer_1*input_layer); 
end
if isempty(mult2)
       mult2=zeros(layer_2,layer_1*layer_2); 
end
if isempty(mult3)
       mult3=zeros(layer_3,layer_2*layer_3); 
end
if isempty(vy)
       vy=zeros(input_layer,M); 
end

if memory_alloc_flag==0
 %write memory allocation for looped code here.It runs once and store it in memory.  
 mult1=[];
 mult2=[];
 mult3=[];
  for iteration =1:layer_1
   mult1=[mult1;[zeros(1,(iteration-1)*input_layer) ones(1,input_layer) zeros(1,(layer_1-iteration)*input_layer)]];
  end
  for iterate=1:layer_2
   mult2=[mult2;[zeros(1,(iterate-1)*layer_1) ones(1,layer_1) zeros(1,(layer_2-iterate)*layer_1)]];
  end
  for iterate=1:layer_3
   mult3=[mult3;[zeros(1,(iterate-1)*layer_2) ones(1,layer_2) zeros(1,(layer_3-iterate)*layer_2)]];
  end
 
 for k= 1:input_layer
    for j = 1:M 
        if k<=(M/2)+1 && k>=1
            vy(k,j)=(1/M)*cos(pi*(M-j)*(k-1)/(M/2));
        elseif k<=M && k>=(M/2)+1
            vy(k,j)=-(1/M)*sin(pi*(M-j)*(k-1)/(M/2));
        elseif k>M
            vy(k,j)=0;     
        end
    end
 end
 memory_alloc_flag=1; 
end

%%
%============All other Initiaisation =========================>

%Initialisation of delta of weight storage
if isempty(del_w1)
    del_w1=zeros(1,input_layer*layer_1);
end
if isempty(del_w2)
    del_w2=zeros(1,layer_2*layer_1);
end
if isempty(del_w3)
    del_w3=zeros(1,layer_2*layer_3);
end

%Intialising iteration number & cost value. 
if isempty(itr)
    itr=0;
end
if isempty(J)
    J=0;
end


%gradient initialisation(in matrix form)
if isempty(g1)
    g1= zeros(M,input_layer*layer_1);   
end
if isempty(g2)
    g2= zeros(M,layer_1*layer_2);   
end
if isempty(g3)
    g3= zeros(M,layer_3*layer_2);   
end

%%
%Input vector creation code block
%x_in = [real(u1(1:(size(u1,2)/2)+1)) imag(u1(1:(size(u1,2)/2)-1))];
%v=transpose([x_in transpose(u2)]);

v=transpose([u1' transpose(u2)]);

%%
%RBNN core vectorised algorithm implementation 

%--------------->forward propogation ------------>

z1=w1'*v ;
%a1=(1./(1+exp(-z1)));
%an1=(a1-0.5);
a1=max(z1,0)+0.1*min(0,z1);
z2=w2'*a1 ;
%z2=w2'*an1 ;
%a2=(1./(1+exp(-z2)));
%an2=(a2-0.5);
a2=max(z2,0)+0.1*min(0,z2);
%z3=w3'*an2 ;
z3=w3'*a2 ;
a3=(1./(1+exp(-z3)));
an3=(a3-0.5)*10;

%-------------> Backward Propogation -------->

%calculation of Nv:
da3_z3=a3.*(1-a3)*10;
dn_a2=w3'.*repmat(da3_z3,1,layer_2);
%da2_z2=a2.*(1-a2);
da2_z2=(1*(a2>=0) + 0.1*((a2>=0)==0));
dn_z2= dn_a2.* repmat(transpose(da2_z2),output_layer,1);
dn_a1=dn_z2*w2';
%da1_z1=a1.*(1-a1); 
da1_z1=(1*(a1>=0) + 0.1*((a1>=0)==0));
dn_z1=dn_a1.*repmat(transpose(da1_z1),output_layer,1);
dn_v=dn_z1*w1';   %"This is Nv" 

%calculation of aD, A & B 
aD=transpose(F)*dn_v*vy;
A=[aD;eye(M-1) zeros(M-1,1)];
B=[transpose(F) ; zeros(M-1,size(F,1))]; 

%calculation of Nw(diff of N(v,w) wrt each weights)
dIn_3= da3_z3*transpose(a2);
dn_w3=repmat(dIn_3,1,layer_3).* mult3;

dIn_2= da2_z2*transpose(a1);
da2_w2=repmat(dIn_2,1,layer_2).* mult2;
dn_w2=dn_a2*da2_w2;

dIn_1= da1_z1*transpose(v);
da1_w1= repmat(dIn_1,1,layer_1).*mult1;
dn_w1=dn_a1*da1_w1;

%gradient updation
g3=A*g3+B*dn_w3;
g2=A*g2+B*dn_w2;
g1=A*g1+B*dn_w1;

%Training & updation only once in a batch(batch size=M,n=Overall counter) 
if mod(n,M)==0 && stop==0
    del_w1 =alpha*df*1*g1/M ;
    del_w2 =alpha*df*1*g2/M ;
    del_w3 =alpha*df*1*g3/M ;
    del_w_reshaped1= reshape(del_w1,[input_layer,layer_1]);
    del_w_reshaped2= reshape(del_w2,[layer_1,layer_2]);
    del_w_reshaped3= reshape(del_w3,[layer_2,layer_3]);
    w1=w1+ del_w_reshaped1;
    w2=w2+ del_w_reshaped2;
    w3=w3+ del_w_reshaped3; 
    itr=itr+1;
    J= sum(df.^2,'all')/(2*M);
end

%For logging & visulisation purpose
cost=J;
weights=w1;
z1_out=z1;
z2_out=z2;
z3_out=z3;

%NN output assignment
nn_op=an3;


end

== matlab function MIMO/buffer_of_op_fft1 ==
  data: output_fft output size=[1,4]; output_difference_vector output size=[1,4]; dif_ip input; rbnn_output input
function [output_fft,output_difference_vector] = difBuffer(dif_ip,rbnn_output)                      

 sz=4;                       % size of the dft 
 
 persistent a;
 persistent b;
 if isempty(b)
  b= zeros(1,sz);
 end
 if isempty(a)
  a= zeros(1,sz);
 end
 
 
  a= circshift(a,1);
  a(1)=dif_ip;
  b= circshift(b,1);
  b(1)=rbnn_output;

 output_difference_vector=a; 
 output_fft=1/sz*fft(b); 
end

== matlab function MIMO/software_rezonator ==
  data: signalz input; reconstructed_signal output; Fn output size=8
function [reconstructed_signal,Fn]   = rezonator(signalz)

persistent numberofrezonator;
persistent g c bfr_rezo_sm aft_delay dft_out;
persistent out signal_dif;
persistent n;
persistent memory_alloc_flag;


%assign the number of rezonator here. For configuring it for higher order
%rezonator  we need to change (1) 'numberofrezonaotor' variable
if isempty(numberofrezonator)
        numberofrezonator = 8;   %here 16 parallel rezonators
end
N=8;
%Initialisation of memory allocations/variables ====> 
if isempty(memory_alloc_flag)
        memory_alloc_flag = 0; 
end
if isempty(g)
       g=zeros(numberofrezonator,numberofrezonator,'like',0i); 
end
if isempty(c)
       c=zeros(numberofrezonator,numberofrezonator,'like',0i); 
end
if memory_alloc_flag==0
 for i=0:numberofrezonator-1
  for j= 0:numberofrezonator-1
   g(i+1,j+1)=1/numberofrezonator*(exp(-1i*2*pi*i*j/numberofrezonator));
   c(i+1,j+1)=(exp(1i*2*pi*i*j/numberofrezonator));
  end 
 end
 memory_alloc_flag=1;
end


%Initialisation of variables  =====> 
if isempty(n)
        n = 0;   
end 
if isempty(out)
  out=0+0i;
end
if isempty(signal_dif)
  signal_dif=0+0i;
end
if isempty(bfr_rezo_sm)
  bfr_rezo_sm=repmat(0+0i,numberofrezonator,1);
end
if isempty(aft_delay)
  aft_delay=repmat(0+0i,numberofrezonator,1);
end
if isempty(dft_out)
  dft_out=repmat(0+0i,numberofrezonator,1);
end

%creating cycle of rotation for selection of correct column of g & c.
cycle=mod(n,numberofrezonator);

%resonator core -----------------------------> 
dft_out=c(:,cycle+1).*aft_delay;
out= sum(dft_out,1);
signal_dif=signalz-out;
bfr_rezo_sm=g(:,cycle+1).*signal_dif;

%counting the counter
n=n+1;

% output assignment ------------------>
reconstructed_signal=out;
dft=aft_delay; 
%N=size(dft,1);
a=1:1:N/2-1;
b=N/2+1:1:N-1;
dft_trans=transpose(dft);
Fn=5*transpose([real(dft_trans(1)) 2*(real(dft_trans(2:N/2)).*cos(2*pi*a*n/N)-imag(dft_trans(2:N/2)).*sin(2*pi*a*n/N)) -1^n*real(dft_trans(N/2+1)) -2*(imag(dft_trans(N/2+2:N)).*cos(2*pi*b*n/N)+real(dft_trans(N/2+2:N)).*sin(2*pi*b*n/N))]);
%--------output assignment over----------<

%final updation of buffer ------>>>>>>>>>>>>
aft_delay= aft_delay+bfr_rezo_sm; 
end

== matlab function MIMO/RBNN_output ==
  data: dft input; yn output; freq_char input
function yn = fcn(dft,freq_char)
yn=transpose(freq_char)*dft;
end

== matlab function MIMO/RBNN_output1 ==
  data: dft input; yn output; freq_char input
function yn = fcn(dft,freq_char)
yn=transpose(freq_char)*dft;
end
